simulink model "mass_spring_damper"  (R2017b)
settings: Solver=VariableStepAuto  StartTime=0.0  StopTime=10.0  RelTol=1e-3
undefined symbols (not defined in the file): c, k, m
settings Model: Creator=jc2182  LastModifiedBy=jc2182

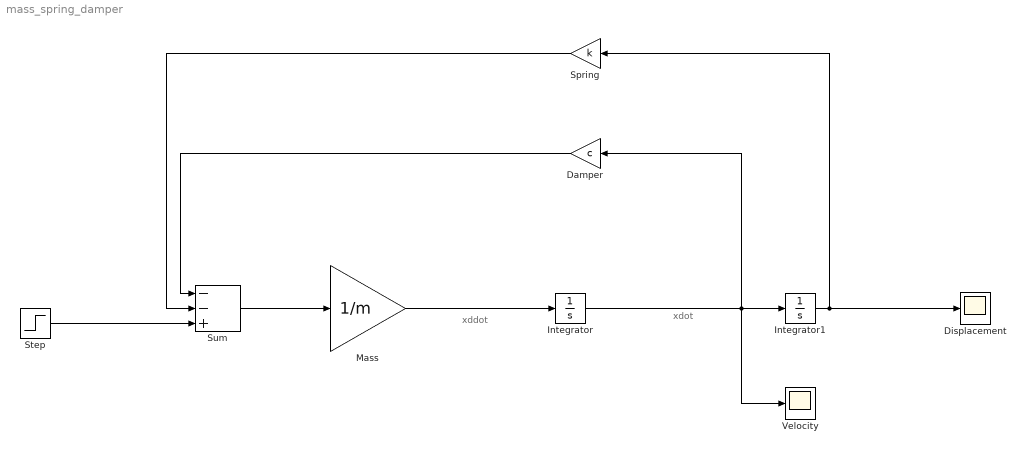
== system mass_spring_damper ==
  note: xdot
  note: xddot
  Damper : Gain  Gain=c
  Displacement : Scope
  Integrator : Integrator
  Integrator1 : Integrator
  Mass : Gain  Gain=1/m
  Spring : Gain  Gain=k
  Step : Step  After=1000  SampleTime=0
  Sum : Sum  Inputs=--+
  Velocity : Scope
  wires:
  Mass/1 -> Integrator/1
  Integrator/1 -> Velocity/1, Damper/1, Integrator1/1
  Integrator1/1 -> Displacement/1, Spring/1
  Sum/1 -> Mass/1
  Damper/1 -> Sum/1
  Spring/1 -> Sum/2
  Step/1 -> Sum/3
